simulink model "Pojednostavljeni_model_backstepping"  (R2020b)
settings: Solver=ode4  StartTime=0.0  StopTime=1000  FixedStep=0.01  RelTol=1e-3
model workspace (MAT data in the model file):
  D1 = 0
  D2 = 0
  D3 = 0
  Kd1 = 0
  Kd2 = 0
  Kd3 = 0
  Kp1 = 0
  Kp2 = 0
  Kp3 = 0
undefined symbols (not defined in the file): B, D, E_c, gama_c, gama_vjet, H, Iz, KD1, KD2, KD3, KP1, KP2, KP3, Kurs_poc, L, La1, La2, La3, m, N_c, Nr, Nrdot, Nv, Polozaj_poc_E, Polozaj_poc_N, r_o, ro, ro_vj, Sig, T, V_c, V_vj, Xu, Xudot, Yr, Yrdot, Yv, Yvdot
libraries: simulink_extras x9, simulink x2
settings Model: Creator=Luka  LastModifiedBy=Luka
settings SolverCC: AlgebraicLoopSolver=LineSearch

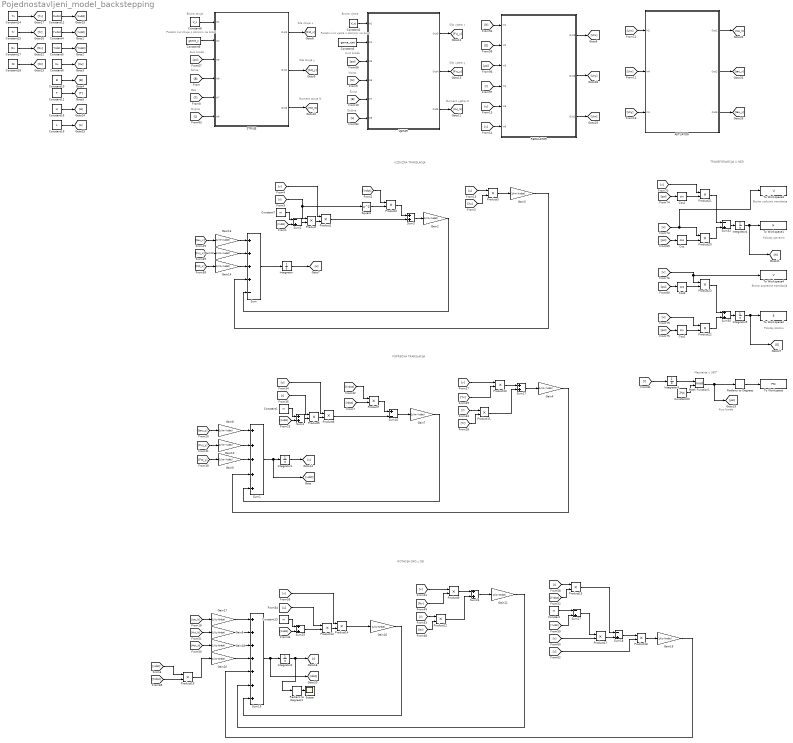
== system Pojednostavljeni_model_backstepping ==
  note: Mapiranje u 360°
  note: Duljina
  note: Visina
  note: Gaz
  note: Širina
  note: Kurs broda
  note: Sila struje x
  note: Kurs broda
  note: Pocetni kut struje s obzirom na brod
  note: Brzina struje
  note: Brzina vjetra
  note: Pocetni kut vjetra s obzirom na brod
  note: Kurs broda
  note: Sila vjetra x
  note: Sila vjetra y
  note: Moment vjetra N
  note: Sila struje y
  note: Moment struje N
  note: UZDUŽNA TRANSLACIJA
  note: POPREČNA TRANSLACIJA
  note: ROTACIJA OKO z OSI
  note: TRANSFORAMCIJA U NED
  note: Položaj istočno
  note: Položaj sjeverno
  note: Brzina uzdužna translacija
  note: Brzina poprečna translacija
  note: Širina
  note: Duljina
  AKTUATOR : Subsystem
  Constant{,1,7,13} (4 alike) : Constant  Value=m
  Constant10 : Constant  Value=B
  Constant11 : Constant  Value=T
  Constant12 : Constant  Value=Xudot
  Constant14 : Constant  Value=Yv
  Constant15 : Constant  Value=Yr
  Constant16 : Constant  Value=H
  Constant17 : Constant  Value=Nv
  Constant18 : Constant  Value=Nr
  Constant19 : Constant  Value=L
  Constant2 : Constant  Value=V_vj
  Constant20 : Constant  Value=2*pi
  Constant3 : Constant  Value=gama_vjet
  Constant4 : Constant  Value=Yvdot
  Constant5 : Constant  Value=Yrdot
  Constant6 : Constant  Value=Xu
  Constant8 : Constant  Value=V_c
  Constant9 : Constant  Value=gama_c
  Cos : Trigonometry  Operator=cos
  Cos1 : Trigonometry
  Cos2 : Trigonometry
  Cos3 : Trigonometry  Operator=cos
  Gain{4,7..10} (5 alike) : Gain  Gain=1/(m-Yvdot)
  Gain{5,11,16..20} (7 alike) : Gain  Gain=1/(Iz-Nrdot)
  Gain{2..3,12..14} (5 alike) : Gain  Gain=1/(m-Xudot)
  Integrator : Integrator
  Integrator1 : Integrator
  Integrator2 : Integrator
  Integrator3 : Integrator  InitialCondition=Kurs_poc
  Integrator4 : Integrator  InitialCondition=Polozaj_poc_N
  Integrator5 : Integrator  InitialCondition=Polozaj_poc_E
  Math Function1 : Math  Operator=mod  SaturateOnIntegerOverflow=on
  Product{,1..3,5..7,9..15,17..23} (21 alike) : Product
  REGULATOR : Subsystem
  Radians to Degrees : simulink_extras/Transformations/Radians to Degrees
  Radians to Degrees1 : simulink_extras/Transformations/Radians to Degrees
  STRUJE : Subsystem
  Scope : Scope
  Square : Math  Operator=square  SaturateOnIntegerOverflow=on
  Sum : Sum  Inputs=++++-
  Sum1 : Sum  Inputs=+++++
  Sum10 : Sum  Inputs=+-
  Sum15 : Sum  Inputs=+++++++
  Sum{3..4,17,24..25,35} (6 alike) : Sum
  Sum{2,18,27,32} (4 alike) : Sum  Inputs=-+
  To Workspace : ToWorkspace  VariableName=PSI  SaveFormat=Timeseries  SampleTime=-1
  To Workspace1 : ToWorkspace  VariableName=N  SaveFormat=Timeseries  SampleTime=-1
  To Workspace2 : ToWorkspace  VariableName=E  SaveFormat=Timeseries  SampleTime=-1
  To Workspace3 : ToWorkspace  VariableName=U  SaveFormat=Timeseries  SampleTime=-1
  To Workspace4 : ToWorkspace  VariableName=V  SaveFormat=Timeseries  SampleTime=-1
  VJETAR : Subsystem
  wires:
  Constant2/1 -> VJETAR/1(In1)
  Constant3/1 -> VJETAR/2(In2)
  [psi] -> VJETAR/3(In5)
  VJETAR/1(Out3) -> [Fvj_x]
  VJETAR/2(Out4) -> [Fvj_y]
  VJETAR/3(Out5) -> [Mvj_N]
  Sum/1 -> Integrator/1
  Constant4/1 -> [Yvdot]
  Constant5/1 -> [Yrdot]
  Constant6/1 -> [Xu]
  Constant7/1 -> Sum2/1
  Sum2/1 -> Product/2
  [r] -> Square/1, Product/1
  [Yvdot] -> Sum2/2
  Constant8/1 -> STRUJE/1(In1)
  [psi] -> STRUJE/3(In5)
  Constant10/1 -> [B]
  Constant11/1 -> [T]
  [B] -> STRUJE/4(In6)
  [T] -> STRUJE/5(In7)
  [H] -> VJETAR/4(In6)
  [B] -> VJETAR/5(In7)
  Product/1 -> Product1/2
  Product1/1 -> Sum3/2
  Square/1 -> Product2/2
  [Yrdot] -> Product2/1
  Product2/1 -> Sum3/1
  Integrator/1 -> [u]
  [v] -> Product1/1
  [u] -> Product3/1
  [Xu] -> Product3/2
  Gain2/1 -> Sum/5
  [Fst_y] -> Gain9/1
  Gain7/1 -> Sum1/5
  Product6/1 -> Sum10/2
  Gain10/1 -> Sum1/2
  Sum10/1 -> Gain7/1
  Product5/1 -> Product6/2
  [r] -> Product5/1
  [Yrdot] -> Product7/1
  [Fvj_y] -> Gain10/1
  [u] -> Product6/1
  Product7/1 -> Sum10/1
  Gain9/1 -> Sum1/3
  Gain8/1 -> Sum1/1
  Integrator1/1 -> [v]
  [Xudot] -> Sum4/2
  Constant1/1 -> Sum4/1
  Sum4/1 -> Product5/2
  Product3/1 -> Gain3/1
  Gain13/1 -> Sum/1
  Gain12/1 -> Sum/2
  Gain14/1 -> Sum/3
  [Fvj_x] -> Gain12/1
  Sum3/1 -> Gain2/1
  Constant12/1 -> [Xudot]
  [rdot] -> Product7/2
  [v] -> Product10/1
  [Yv] -> Product10/2
  Product10/1 -> Sum17/1
  [r] -> Product11/1
  [Yr] -> Product11/2
  Product11/1 -> Sum17/2
  Constant14/1 -> [Yv]
  Constant15/1 -> [Yr]
  Gain4/1 -> Sum1/4
  Gain16/1 -> Sum15/7
  Gain18/1 -> Sum15/3
  [Mvj_N] -> Gain5/1
  Product14/1 -> Gain16/1
  Gain11/1 -> Sum15/6
  Integrator2/1 -> Radians to Degrees1/1, [r]
  Product12/1 -> Sum24/2
  [r] -> Product12/1
  Gain5/1 -> Sum15/2
  [Nr] -> Product12/2
  Sum25/1 -> Product13/2
  [Xudot] -> Sum25/2
  Constant13/1 -> Sum25/1
  Gain17/1 -> Sum15/1
  [v] -> Product9/1
  [Nv] -> Product9/2
  [u] -> Product13/1
  Product9/1 -> Sum24/1
  Sum15/1 -> Integrator2/1, [rdot]
  [Mst_N] -> Gain18/1
  Product13/1 -> Product14/2
  [v] -> Product14/1
  Constant17/1 -> [Nv]
  Constant18/1 -> [Nr]
  [r] -> Product15/1
  [Yrdot] -> Product15/2
  Product15/1 -> Sum18/1
  Constant/1 -> Sum27/1
  [Yvdot] -> Sum27/2
  [v] -> Product17/2
  Sum27/1 -> Product17/1
  Product17/1 -> Sum18/2
  Sum18/1 -> Product18/1
  Product18/1 -> Gain19/1
  Gain19/1 -> Sum15/5
  [Yrdot] -> Product19/2
  [vdot] -> Product19/1
  Product19/1 -> Gain20/1
  Gain20/1 -> Sum15/4
  Product20/1 -> Sum32/2
  [psi] -> Cos/1
  Cos/1 -> Product20/2
  [u] -> To Workspace3/1, Product20/1
  Cos1/1 -> Product21/2
  [psi] -> Cos1/1
  [v] -> Product21/1
  Product21/1 -> Sum32/1
  Sum32/1 -> Integrator4/1
  Integrator4/1 -> [N], To Workspace1/1
  Cos3/1 -> Product23/2
  Product22/1 -> Sum35/2
  Product23/1 -> Sum35/1
  [u] -> Product22/1
  [psi] -> Cos2/1
  Sum35/1 -> Integrator5/1
  Cos2/1 -> Product22/2
  [psi] -> Cos3/1
  [r] -> Integrator3/1
  [v] -> Product23/1, To Workspace4/1
  Constant9/1 -> STRUJE/2(In2)
  Constant16/1 -> [H]
  Constant19/1 -> [L]
  [L] -> VJETAR/6(In8)
  [L] -> STRUJE/6(In8)
  Integrator5/1 -> [E], To Workspace2/1
  Radians to Degrees/1 -> To Workspace/1
  Sum17/1 -> Gain4/1
  Sum1/1 -> [vdot], Integrator1/1
  Sum24/1 -> Gain11/1
  [u] -> Product18/2
  Integrator3/1 -> Math Function1/1
  Constant20/1 -> Math Function1/2
  Math Function1/1 -> [psi], Radians to Degrees/1
  [Fst_x] -> Gain14/1
  STRUJE/1(Out3) -> [Fst_x]
  STRUJE/2(Out4) -> [Fst_y]
  STRUJE/3(Out5) -> [Mst_N]
  [tau_x] -> Gain13/1
  [tau_N] -> Gain17/1
  Gain3/1 -> Sum/4
  [tau_y] -> Gain8/1
  AKTUATOR/3(Out6) -> [tau_y]
  AKTUATOR/1(Out1) -> [tau_N]
  [Urn] -> AKTUATOR/1(In2)
  [Urx] -> AKTUATOR/2(In4)
  [E] -> REGULATOR/2(In2)
  REGULATOR/2(Out5) -> [Ury]
  [psi] -> REGULATOR/3(In3)
  [r] -> REGULATOR/4(In4)
  [N] -> REGULATOR/1(In1)
  REGULATOR/1(Out3) -> [Urx]
  AKTUATOR/2(Out2) -> [tau_x]
  [u] -> REGULATOR/5(In5)
  [v] -> REGULATOR/6(In6)
  REGULATOR/3(Out1) -> [Urn]
  [Ury] -> AKTUATOR/3(In1)
  Radians to Degrees1/1 -> Scope/1

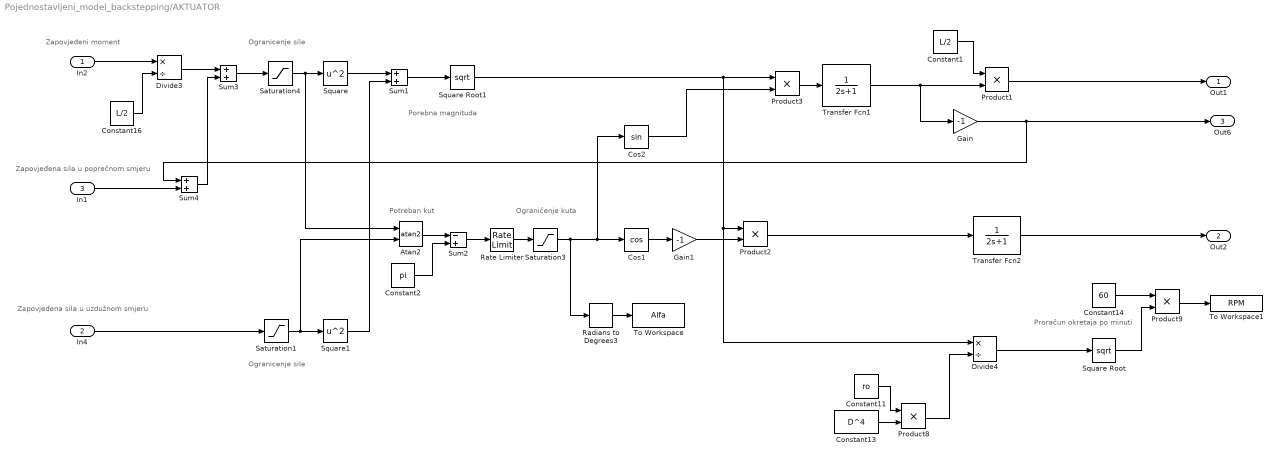
== system Pojednostavljeni_model_backstepping/AKTUATOR ==
  note: Zapovjeđena sila u poprečnom smjeru
  note: Porebna magnituda
  note: Zapovjeđeni moment
  note: Zapovjeđena sila u uzdužnom smjeru
  note: Proračun okretaja po minuti
  note: Ograničenje kuta
  note: Ogranicenje sile
  note: Potreban kut
  note: Ogranicenje sile
  In2 : Inport
  In4 : Inport  Port=2
  In1 : Inport  Port=3
  Atan2 : Trigonometry  Operator=atan2
  Constant1 : Constant  Value=L/2
  Constant11 : Constant  Value=ro
  Constant13 : Constant  Value=D^4
  Constant14 : Constant  Value=60
  Constant16 : Constant  Value=L/2
  Constant2 : Constant  Value=pi
  Cos1 : Trigonometry  Operator=cos
  Cos2 : Trigonometry
  Divide3 : Product  Inputs=*/
  Divide4 : Product  Inputs=*/
  Gain : Gain  Gain=-1
  Gain1 : Gain  Gain=-1
  Product{1..3,8..9} (5 alike) : Product
  Radians to Degrees3 : simulink_extras/Transformations/Radians to Degrees
  Rate Limiter : RateLimiter  RisingSlewLimit=40*pi/180  FallingSlewLimit=-40*pi/180  SampleTimeMode=inherited
  Saturation1 : Saturate  UpperLimit=300  LowerLimit=0
  Saturation3 : Saturate  UpperLimit=250*pi/180  LowerLimit=110*pi/180
  Saturation4 : Saturate  UpperLimit=280  LowerLimit=-280
  Square : Math  Operator=square  SaturateOnIntegerOverflow=on
  Square Root : Sqrt  SaturateOnIntegerOverflow=on
  Square Root1 : Sqrt  SaturateOnIntegerOverflow=on
  Square1 : Math  Operator=square  SaturateOnIntegerOverflow=on
  Sum1 : Sum
  Sum2 : Sum  Inputs=-+
  Sum3 : Sum
  Sum4 : Sum
  To Workspace : ToWorkspace  VariableName=Alfa  SaveFormat=Timeseries  SampleTime=-1
  To Workspace1 : ToWorkspace  VariableName=RPM  SaveFormat=Timeseries  SampleTime=-1
  Transfer Fcn1 : TransferFcn  Denominator=[2 1]
  Transfer Fcn2 : TransferFcn  Denominator=[2 1]
  Out1 : Outport
  Out2 : Outport  Port=2
  Out6 : Outport  Port=3
  wires:
  Sum2/1 -> Rate Limiter/1
  Product8/1 -> Divide4/2
  Gain/1 -> Sum4/1, Out6/1
  Sum1/1 -> Square Root1/1
  Constant16/1 -> Divide3/2
  Saturation3/1 -> Cos2/1, Cos1/1, Radians to Degrees3/1
  Saturation4/1 -> Atan2/1, Square/1
  Divide3/1 -> Sum3/1
  Cos1/1 -> Gain1/1
  Gain1/1 -> Product2/2
  In4/1 -> Saturation1/1
  Constant11/1 -> Product8/1
  Rate Limiter/1 -> Saturation3/1
  Transfer Fcn1/1 -> Gain/1, Product1/2
  Square1/1 -> Sum1/2
  Square/1 -> Sum1/1
  Product3/1 -> Transfer Fcn1/1
  Cos2/1 -> Product3/2
  Atan2/1 -> Sum2/1
  In2/1 -> Divide3/1
  Product2/1 -> Transfer Fcn2/1
  Product9/1 -> To Workspace1/1
  Product1/1 -> Out1/1
  Square Root/1 -> Product9/2
  Transfer Fcn2/1 -> Out2/1
  Constant13/1 -> Product8/2
  Divide4/1 -> Square Root/1
  Square Root1/1 -> Divide4/1, Product2/1, Product3/1
  Saturation1/1 -> Atan2/2, Square1/1
  Radians to Degrees3/1 -> To Workspace/1
  Constant2/1 -> Sum2/2
  Constant1/1 -> Product1/1
  Constant14/1 -> Product9/1
  Sum3/1 -> Saturation4/1
  In1/1 -> Sum4/2
  Sum4/1 -> Sum3/2

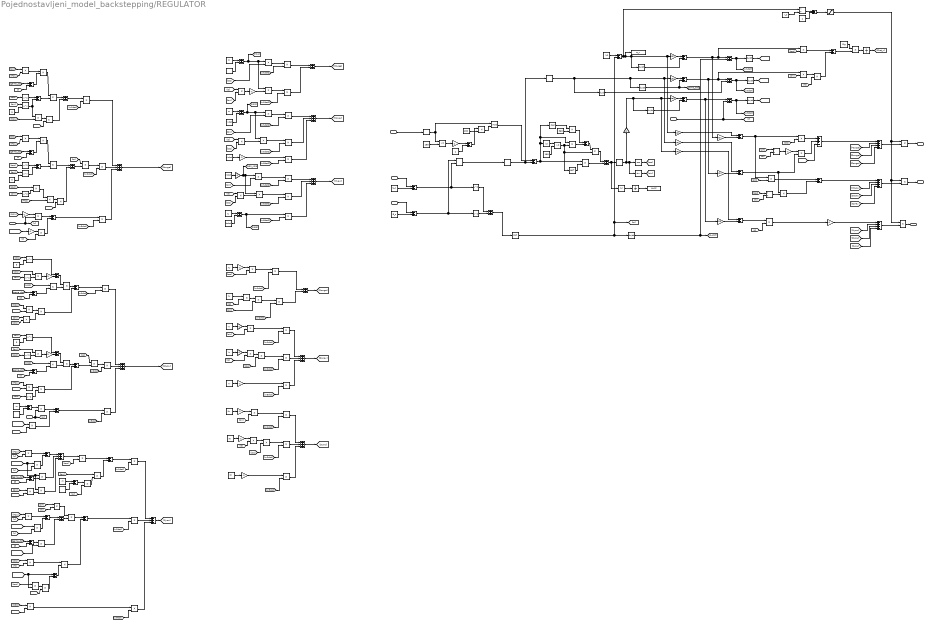
== system Pojednostavljeni_model_backstepping/REGULATOR ==
  note: Integralno djelovanje u napredovanju
  note: Zapovjeđeni moment
  note: Dx33
  note: Dx32
  note: Dx31
  note: Dx12
  note: Dx11
  note: Cx32
  note: Cx31
  note: Cx13
  note: Cx21
  note: v
  note: u
  note: Cx11
  note: Mx11
  note: xr1dot
  note: r
  note: z13dot
  note: z12dot
  note: z11dot
  note: x1dot
  note: z13
  note: z11
  note: x1d
  note: Kurs u +/- 180°(x3)
  note: Udaljenost od centra kruznice (x1)
  note: Pogreška kuta -/+ 180
  note: Zapovjeđena sila u uzdužnom smjeru
  note: Zapovjeđena sila u poprečnom smjeru
  note: Kurs broda
  note: Potreban kurs broda +/- 180
  note: Polozaj N
  note: Polozaj E
  note: Polozaj kruznice N
  note: Polozaj kruznice E
  note: z12
  note: x3dot
  note: x2dot
  note: z21
  note: z22
  note: z23
  note: xr2dot
  note: xr3dot
  note: xr1dot2
  note: xr2dot2
  note: xr3dot2
  note: Mx12
  note: Mx21
  note: Mx22
  note: Mx23
  note: Mx31
  note: Mx32
  note: Mx33
  note: Cx12
  note: Cx22
  note: Cx23
  note: Cx33
  note: Dx21
  note: Dx22
  note: Dx23
  note: Ublažavanje regulacije u slučaju da je brod unutar kružnice
  In1 : Inport
  In2 : Inport  Port=2
  In3 : Inport  Port=3
  In4 : Inport  Port=4
  In5 : Inport  Port=5
  In6 : Inport  Port=6
  Abs : Abs
  Abs3 : Abs
  Atan2 : Trigonometry  Operator=atan2
  Constant : Constant  Value=r_o
  Constant1 : Constant  Value=N_c
  Constant10 : Constant  Value=Yrdot
  Constant12 : Constant  Value=Iz
  Constant13 : Constant  Value=Nrdot
  Constant14 : Constant  Value=180
  Constant{15..16,19..20} (4 alike) : Constant  Value=3
  Constant17 : Constant  Value=180
  Constant18 : Constant
  Constant2 : Constant  Value=E_c
  Constant{3,6,21,23} (4 alike) : Constant  Value=m
  Constant22 : Constant  Value=Xudot
  Constant24 : Constant  Value=Xudot
  Constant25 : Constant  Value=180
  Constant26 : Constant  Value=Xu
  Constant27 : Constant  Value=360
  Constant28 : Constant  Value=Xu
  Constant29 : Constant  Value=Yv
  Constant30 : Constant  Value=Yv
  Constant31 : Constant  Value=Yr
  Constant32 : Constant  Value=Nv
  Constant33 : Constant  Value=Nv
  Constant34 : Constant  Value=Nr
  Constant39 : Constant  Value=r_o
  Constant4 : Constant  Value=Xudot
  Constant40 : Constant
  Constant5 : Constant  Value=Sig
  Constant7 : Constant  Value=Yvdot
  Constant9 : Constant  Value=Yrdot
  Cos : Trigonometry  Operator=cos
  Degrees to Radians : simulink_extras/Transformations/Degrees to Radians
  Degrees to Radians1 : simulink_extras/Transformations/Degrees to Radians
  Derivative{,1..7} (8 alike) : Derivative
  Divide : Product  Inputs=*/
  Divide1 : Product  Inputs=*/
  Divide2 : Product  Inputs=*/
  Gain : Gain  Gain=La1
  Gain1 : Gain  Gain=La3
  Gain{7..11,14..20,24,27..28} (15 alike) : Gain  Gain=-1
  Gain12 : Gain  Gain=3
  Gain13 : Gain  Gain=3
  Gain2 : Gain  Gain=La2
  Gain21 : Gain  Gain=KD1
  Gain22 : Gain  Gain=KD3
  Gain23 : Gain  Gain=KD2
  Gain3 : Gain  Gain=KP1
  Gain4 : Gain  Gain=KP3
  Gain5 : Gain  Gain=2
  Gain6 : Gain  Gain=KP2
  GreaterThan : RelationalOperator  OutDataTypeStr=boolean  RndMeth=Simplest
  GreaterThan1 : RelationalOperator  OutDataTypeStr=boolean  RndMeth=Simplest
  Integrator : Integrator
  Integrator1 : Integrator
  Mod2 : Math  Operator=mod  SaturateOnIntegerOverflow=on
  NOT : Logic  Operator=NOT  IconShape=distinctive  AllPortsSameDT=off  OutDataTypeStr=boolean
  Power{,1..3} (4 alike) : Math  Operator=pow  SaturateOnIntegerOverflow=on
  Product{,1..102,104..106} (106 alike) : Product
  Radians to Degrees : simulink_extras/Transformations/Radians to Degrees
  Radians to Degrees2 : simulink_extras/Transformations/Radians to Degrees
  Saturation : Saturate  UpperLimit=1  LowerLimit=0
  Sign : Signum
  Sin : Trigonometry
  Sqrt : Sqrt  SaturateOnIntegerOverflow=on
  Square{,1..7} (8 alike) : Math  Operator=square  SaturateOnIntegerOverflow=on
  Sum{,1,5,7..10,14,17,29,32,43,59} (13 alike) : Sum  Inputs=-+
  Sum{11..13,20..22,24..26,28,31,36..37,39,41..42,44} (17 alike) : Sum  Inputs=+-
  Sum{2..4,6,15,18,23,30,33,35,40,45..46,48,51..53,55,64} (19 alike) : Sum
  Sum{16,19,27,34,47,49..50} (7 alike) : Sum  Inputs=+++
  Sum38 : Sum  Inputs=+-+
  Sum54 : Sum  Inputs=++-
  Sum56 : Sum  Inputs=++++
  Sum57 : Sum  Inputs=++++
  Sum58 : Sum  Inputs=++++
  To Workspace : ToWorkspace  VariableName=e_psi  SaveFormat=Timeseries  SampleTime=-1
  To Workspace1 : ToWorkspace  VariableName=e_x  SaveFormat=Timeseries  SampleTime=-1
  Out3 : Outport
  Out5 : Outport  Port=2
  Out1 : Outport  Port=3
  wires:
  Constant1/1 -> Sum/2
  In1/1 -> Sum/1
  Constant2/1 -> Sum1/2
  In2/1 -> Sum1/1
  Sum1/1 -> Square/1, Atan2/1
  Sum/1 -> Square1/1, Atan2/2
  Square1/1 -> Sum2/1
  Square/1 -> Sum2/2
  Sum2/1 -> Sqrt/1
  Atan2/1 -> Radians to Degrees2/1
  Radians to Degrees2/1 -> Degrees to Radians1/1, Sum8/2
  Constant18/1 -> Sum14/2
  Gain5/1 -> Sum14/1
  Radians to Degrees/1 -> GreaterThan/1, Mod2/1
  Constant17/1 -> GreaterThan/2
  GreaterThan/1 -> Gain5/1
  Sum14/1 -> Product10/1
  Mod2/1 -> Sum8/1
  Constant14/1 -> Product10/2
  Product10/1 -> Mod2/2
  Abs3/1 -> GreaterThan1/1
  Constant25/1 -> GreaterThan1/2
  GreaterThan1/1 -> Product16/2, NOT/1, Product15/2
  Sum8/1 -> Product15/1, Sign/1, Abs3/1, Product18/1
  Product15/1 -> Sum17/2
  Sum17/1 -> Product16/1
  Product16/1 -> Sum18/1
  Constant27/1 -> Product17/2
  Product17/1 -> Sum17/1
  NOT/1 -> Product18/2
  Product18/1 -> Sum18/2
  Sign/1 -> Product17/1
  Constant/1 -> Sum5/1
  Derivative1/1 -> Sum3/2
  Derivative2/1 -> Sum4/2, [gama_dot]
  Derivative/1 -> [ro_dot], Sum7/2
  Gain/1 -> Sum3/1
  Gain2/1 -> Sum4/1
  Gain1/1 -> Sum6/1
  Sum4/1 -> Gain23/1, Product100/1, Sum9/1
  Sum7/1 -> [xr1dot], Derivative4/1
  Sum9/1 -> [xr2dot], Derivative5/1
  Sum10/1 -> [xr3dot], Derivative6/1
  Constant3/1 -> Sum11/1
  Constant4/1 -> Sum11/2
  Sum11/1 -> [M11], Product1/1, Product3/1
  Cos/1 -> [cos]
  Sin/1 -> [sin]
  [cos] -> Product1/2
  [ro] -> Product2/1
  [sin] -> Product2/2
  Product2/1 -> Gain7/1
  Gain7/1 -> Product3/2
  Constant7/1 -> Sum12/2
  Constant6/1 -> Sum12/1
  Sum12/1 -> [M22], Product6/1, Product4/1
  [sin] -> Product4/2
  [ro] -> Product5/1
  [cos] -> Product5/2
  Product5/1 -> Product6/2
  Constant9/1 -> Gain8/1
  [sin] -> Product7/2
  Constant10/1 -> Gain9/1
  Gain9/1 -> [M32_M23], Product9/1, Product7/1
  [ro] -> Product8/1
  Product8/1 -> Product9/2
  [cos] -> Product8/2
  Constant12/1 -> Sum13/1
  Constant13/1 -> Sum13/2
  Derivative4/1 -> [xr1dot2]
  Derivative5/1 -> [xr2dot2]
  Derivative6/1 -> [xr3dot2]
  Product1/1 -> Product/1
  [xr1dot2] -> Product/2
  Product3/1 -> Product11/1
  [xr2dot2] -> Product11/2
  Product11/1 -> Sum15/2
  Product/1 -> Sum15/1
  Product4/1 -> Product12/1
  [xr1dot2] -> Product12/2
  [xr2dot2] -> Product13/2
  Product6/1 -> Product13/1
  Gain8/1 -> Product14/1
  Product12/1 -> Sum16/1
  Product13/1 -> Sum16/2
  [xr3dot2] -> Product14/2
  Product14/1 -> Sum16/3
  Product7/1 -> Product19/1
  [xr1dot2] -> Product19/2
  Product9/1 -> Product20/1
  [xr2dot2] -> Product20/2
  Sum13/1 -> [M33], Product21/1
  [xr3dot2] -> Product21/2
  Product20/1 -> Sum19/2
  Product21/1 -> Sum19/3
  [sin] -> Product22/1
  [M11] -> Product22/2
  [gama_dot] -> Sum20/1
  In4/1 -> Sum10/2, [r]
  [r] -> Sum20/2
  Product22/1 -> Product23/1
  Sum20/1 -> Product23/2
  [cos] -> Square2/1
  Square2/1 -> Sum21/1
  [sin] -> Power/1
  Constant15/1 -> Power/2
  Power/1 -> Product25/1, Sum21/2
  Sum21/1 -> Product24/2
  Product23/1 -> Product24/1
  Product24/1 -> Sum22/1
  [M11] -> Product25/2
  Product25/1 -> Product26/1
  [ro_dot] -> Product26/2
  Product26/1 -> Sum22/2
  Sum22/1 -> Product27/1
  [xr1dot] -> Product27/2
  Product27/1 -> Sum27/1
  [M11] -> Product31/2
  Product29/1 -> Product30/1
  Product31/1 -> Product32/1
  [sin] -> Power1/1
  [cos] -> Product28/1
  Product28/1 -> Product29/1
  Constant16/1 -> Power1/2
  [r] -> Sum24/2
  Sum25/1 -> Product30/2
  [ro_dot] -> Product32/2
  Sum24/1 -> Product29/2
  [M11] -> Product28/2
  Square3/1 -> Sum25/1
  Product32/1 -> Sum26/2
  [cos] -> Square3/1
  Sum26/1 -> Product34/2
  Power1/1 -> Sum25/2
  Product30/1 -> Sum26/1
  [xr2dot] -> Product33/2
  [gama_dot] -> Sum24/1
  Product33/1 -> Sum27/2
  [ro] -> Product34/1
  Product34/1 -> Product33/1
  [sin] -> Square4/1
  [cos] -> Product35/1
  Square4/1 -> Product35/2
  Product35/1 -> Product31/1
  [M11] -> Gain10/1
  In6/1 -> [v], Product36/2
  Gain10/1 -> Product36/1
  Product36/1 -> Sum23/1
  [M32_M23] -> Gain11/1
  Gain11/1 -> Product37/1
  [r] -> Product37/2
  Product37/1 -> Sum23/2
  [r] -> Sum28/2
  Sum28/1 -> Product38/2
  [gama_dot] -> Sum28/1
  [M22] -> Product38/1
  Product38/1 -> Product39/2
  [cos] -> Product43/1
  Product39/1 -> Sum30/1
  [M22] -> Product40/1
  [ro_dot] -> Product40/2
  Product40/1 -> Product41/1
  Product41/1 -> Sum30/2
  [sin] -> Product42/1
  [cos] -> Product42/2
  Product42/1 -> Product41/2
  [sin] -> Square5/1
  Square5/1 -> Product43/2
  Product43/1 -> Gain12/1
  Gain12/1 -> Sum29/2
  [cos] -> Power2/1
  Constant19/1 -> Power2/2
  Power2/1 -> Sum29/1
  Sum29/1 -> Product39/1
  Sum30/1 -> Product44/1
  [xr1dot] -> Product44/2
  Gain13/1 -> Sum32/2
  Square7/1 -> Product48/2
  [M22] -> Product47/1
  [M22] -> Product45/1
  Power3/1 -> Sum32/1
  Constant20/1 -> Power3/2
  [gama_dot] -> Sum31/1
  Product46/1 -> Sum33/1
  [r] -> Sum31/2
  [xr2dot] -> Product51/2
  [sin] -> Product50/1
  Sum31/1 -> Product45/2
  [ro_dot] -> Product47/2
  Product47/1 -> Product48/1
  Product48/1 -> Sum33/2
  Sum32/1 -> Product46/1
  Product45/1 -> Product46/2
  [sin] -> Power3/1
  Square6/1 -> Product50/2
  Product50/1 -> Gain13/1
  [cos] -> Square7/1
  [cos] -> Square6/1
  Sum33/1 -> Product52/2
  Product52/1 -> Product51/1
  [ro] -> Product52/1
  Product44/1 -> Sum34/1
  Product51/1 -> Sum34/2
  Product49/1 -> Sum27/3
  [xr3dot] -> Product49/2
  Sum23/1 -> Product49/1
  Constant21/1 -> Sum35/1
  Constant22/1 -> Sum35/2
  Sum35/1 -> Product53/1
  In5/1 -> [u], Product53/2
  Product53/1 -> Sum36/1
  [M32_M23] -> Product54/1
  [ro_dot] -> Product54/2
  Product54/1 -> Sum36/2
  Sum36/1 -> Product55/1
  [xr3dot] -> Product55/2
  Product55/1 -> Sum34/3
  [v] -> Product56/2
  [M22] -> Product56/1
  Product56/1 -> Sum37/1
  [r] -> Product57/2
  Product57/1 -> Sum37/2
  Sum37/1 -> Sum38/1
  [cos] -> Product58/2
  [r] -> Sum39/2
  Sum39/1 -> Product59/2
  [gama_dot] -> Sum39/1
  Product59/1 -> Sum38/2
  Sum38/1 -> Product58/1
  [M32_M23] -> Product57/1, Product61/1, Product59/1
  [ro_dot] -> Product60/2
  [sin] -> Product60/1
  Product60/1 -> Product61/2
  Product61/1 -> Sum38/3
  Product58/1 -> Sum40/1
  Product62/1 -> Product63/2
  Constant23/1 -> Sum41/1
  Sum41/1 -> Product62/1
  Constant24/1 -> Sum41/2
  [u] -> Product62/2
  [sin] -> Product63/1
  Product63/1 -> Sum40/2
  Sum40/1 -> Product64/1
  [xr1dot] -> Product64/2
  [sin] -> Product65/1
  Product65/1 -> Product69/1
  [ro] -> Product65/2
  Product66/1 -> Sum42/1
  [v] -> Product66/2
  Product67/1 -> Sum42/2
  Sum42/1 -> Sum43/1
  [M22] -> Product66/1
  [r] -> Product67/2
  [M32_M23] -> Product67/1
  [gama_dot] -> Sum44/1
  [r] -> Sum44/2
  Sum44/1 -> Product68/1
  [M32_M23] -> Product68/2
  Product68/1 -> Sum43/2
  Sum43/1 -> Product69/2
  [ro] -> Product70/2
  [cos] -> Product70/1
  Product69/1 -> Sum45/1
  Product70/1 -> Product71/1
  Product71/1 -> Sum45/2
  [M32_M23] -> Sum46/1, Product72/2
  [cos] -> Product72/1
  [ro_dot] -> Product73/2
  Product72/1 -> Product73/1
  Product73/1 -> Sum46/2
  Sum46/1 -> Product71/2
  Sum45/1 -> Product74/1
  [xr2dot] -> Product74/2
  Product64/1 -> Sum47/1
  Product74/1 -> Sum47/2
  [M33] -> Product75/1
  [ro_dot] -> Product75/2
  [xr3dot] -> Product76/2
  Product75/1 -> Product76/1
  Product76/1 -> Sum47/3
  Constant26/1 -> Gain14/1
  [cos] -> Product77/2
  Gain14/1 -> Product77/1
  Product77/1 -> Product78/1
  [xr1dot] -> Product78/2
  Product78/1 -> Sum48/1
  Constant28/1 -> Product79/1
  [ro] -> Product79/2
  Product79/1 -> Product80/1
  [sin] -> Product80/2
  [xr2dot] -> Product81/2
  Product80/1 -> Product81/1
  Product81/1 -> Sum48/2
  Constant29/1 -> Gain15/1
  Gain15/1 -> Product82/1
  [sin] -> Product82/2
  Product82/1 -> Product83/1
  [xr1dot] -> Product83/2
  Constant30/1 -> Gain16/1
  Gain16/1 -> Product84/1
  [ro] -> Product84/2
  Product84/1 -> Product85/1
  [cos] -> Product85/2
  Product85/1 -> Product86/1
  [xr2dot] -> Product86/2
  Constant31/1 -> Gain17/1
  Gain17/1 -> Product87/1
  [xr3dot] -> Product87/2
  Product83/1 -> Sum49/1
  Product86/1 -> Sum49/2
  Product87/1 -> Sum49/3
  Constant32/1 -> Gain18/1
  [sin] -> Product88/2
  Gain18/1 -> Product88/1
  Product88/1 -> Product89/1
  [xr1dot] -> Product89/2
  Constant33/1 -> Gain19/1
  Gain19/1 -> Product90/1
  [ro] -> Product90/2
  Product90/1 -> Product91/1
  [cos] -> Product91/2
  [xr2dot] -> Product92/2
  Product91/1 -> Product92/1
  Product89/1 -> Sum50/1
  Product92/1 -> Sum50/2
  Constant34/1 -> Gain20/1
  Gain20/1 -> Product93/1
  [xr3dot] -> Product93/2
  Product93/1 -> Sum50/3
  Gain3/1 -> Sum51/1
  Gain21/1 -> Sum51/2
  Gain23/1 -> Sum52/2
  Gain6/1 -> Sum52/1
  Gain22/1 -> Sum53/2
  Gain4/1 -> Sum53/1
  [cos] -> Product94/2
  Sum51/1 -> Product96/1, Product94/1
  Product94/1 -> Sum54/1
  [sin] -> Divide/1
  [ro] -> Divide/2
  Divide/1 -> Gain24/1
  Gain24/1 -> Product95/1
  Sum52/1 -> Product97/1, Product95/2
  Product95/1 -> Sum54/2
  [sin] -> Product96/2
  Product96/1 -> Sum55/1
  [cos] -> Divide1/1
  [ro] -> Divide1/2
  Divide1/1 -> Product97/2
  Product97/1 -> Sum55/2
  Sum53/1 -> Product98/1
  [r] -> Product98/2
  Sum15/1 -> [Msurge]
  Sum16/1 -> [Msway]
  Sum19/1 -> [Myaw]
  Sum48/1 -> [Dsurge]
  Sum49/1 -> [Dsway]
  Sum50/1 -> [Dyaw]
  Sum27/1 -> [Csurge]
  Sum34/1 -> [Csway]
  Sum47/1 -> [Cyaw]
  Sum54/1 -> Sum56/1
  [Msurge] -> Sum56/2
  [Dsurge] -> Sum56/3
  [Csurge] -> Sum56/4
  Sum56/1 -> Product104/2
  Sum55/1 -> Sum57/1
  [Msway] -> Sum57/2
  [Dsway] -> Sum57/3
  [Csway] -> Sum57/4
  Gain27/1 -> Sum58/1
  [Myaw] -> Sum58/2
  [Dyaw] -> Sum58/3
  [Cyaw] -> Sum58/4
  Sum58/1 -> Product106/2
  Derivative7/1 -> Sum9/2
  Derivative3/1 -> Sum6/2
  In3/1 -> Radians to Degrees/1
  Product19/1 -> Sum19/1
  Sum18/1 -> Abs/1, Degrees to Radians/1
  Degrees to Radians1/1 -> Derivative2/1, Gain6/1, Gain2/1, Derivative7/1
  Degrees to Radians/1 -> Cos/1, Sin/1, Gain28/1
  Gain28/1 -> Derivative3/1, Gain1/1, Gain4/1
  Abs/1 -> Integrator/1
  Integrator/1 -> To Workspace/1
  Constant5/1 -> Product99/1
  [sin] -> Product100/2
  [cos] -> Product101/2
  Product100/1 -> Product102/1
  [ro] -> Product102/2
  Product101/1 -> Sum59/1
  Product102/1 -> Sum59/2
  Sum59/1 -> Product99/2
  Product99/1 -> Integrator1/1
  Integrator1/1 -> [Fhat_x]
  [Fhat_x] -> Sum54/3
  Sqrt/1 -> [ro], Sum5/2, Derivative/1
  Sum3/1 -> Sum7/1, Product101/1, Gain21/1
  Sum6/1 -> Sum10/1, Gain22/1
  Product106/1 -> Out1/1
  Product104/1 -> Out3/1
  Sum57/1 -> Product105/2
  Product105/1 -> Out5/1
  Product98/1 -> Gain27/1
  Constant40/1 -> Sum64/2
  Sum64/1 -> Saturation/1
  Divide2/1 -> Sum64/1
  Saturation/1 -> Product104/1, Product106/1, Product105/1
  Sum5/1 -> Divide2/1, Gain/1, Gain3/1, Derivative1/1, To Workspace1/1
  Constant39/1 -> Divide2/2

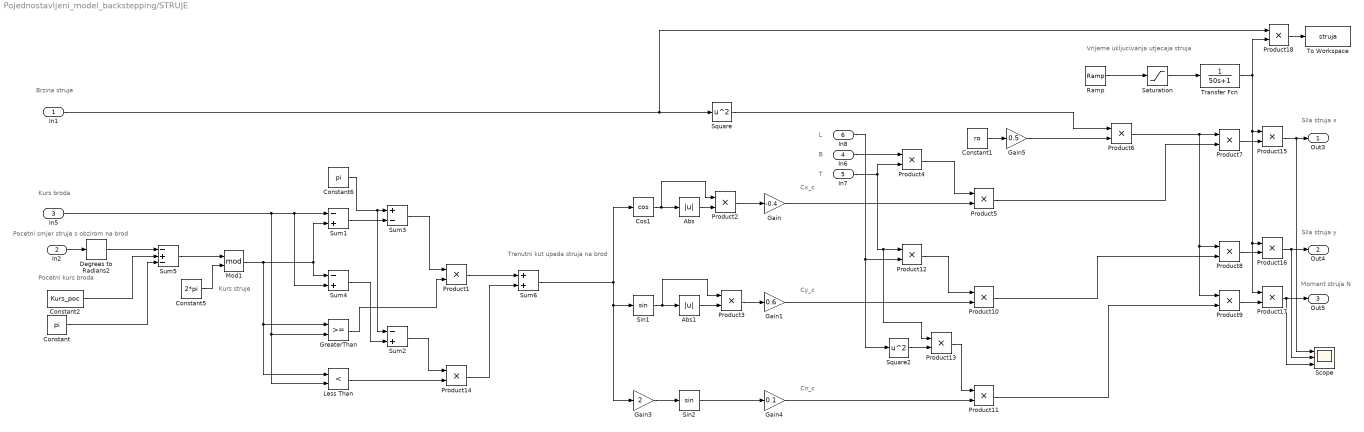
== system Pojednostavljeni_model_backstepping/STRUJE ==
  note: Trenutni kut upada struja na brod
  note: Vrijeme ukljucivanja utjecaja struja
  note: Sila struja x
  note: B
  note: Cx_c
  note: Kurs broda
  note: Pocetni smjer struje s obzirom na brod
  note: Brzina struje
  note: Kurs struje
  note: Cy_c
  note: Cn_c
  note: T
  note: Sila struja y
  note: Moment struja N
  note: L
  note: Pocetni kurs broda
  In1 : Inport
  In2 : Inport  Port=2
  In5 : Inport  Port=3
  In6 : Inport  Port=4
  In7 : Inport  Port=5
  In8 : Inport  Port=6
  Abs : Abs
  Abs1 : Abs
  Constant : Constant  Value=pi
  Constant1 : Constant  Value=ro
  Constant2 : Constant  Value=Kurs_poc
  Constant5 : Constant  Value=2*pi
  Constant6 : Constant  Value=pi
  Cos1 : Trigonometry  Operator=cos
  Degrees to Radians2 : simulink_extras/Transformations/Degrees to Radians
  Gain : Gain  Gain=-0.4
  Gain1 : Gain  Gain=0.6
  Gain3 : Gain  Gain=2
  Gain4 : Gain  Gain=0.1
  Gain5 : Gain  Gain=0.5
  GreaterThan : RelationalOperator  OutDataTypeStr=boolean  RndMeth=Simplest
  Less Than : RelationalOperator  Operator=<  OutDataTypeStr=boolean  RndMeth=Simplest
  Mod1 : Math  Operator=mod  SaturateOnIntegerOverflow=on
  Product{1..18} (18 alike) : Product
  Ramp : simulink/Sources/Ramp  slope=0.002  start=0  InitialOutput=0
  Saturation : Saturate  UpperLimit=1  LowerLimit=-1
  Scope : Scope  NumInputPorts=3
  Sin1 : Trigonometry
  Sin2 : Trigonometry
  Square : Math  Operator=square  SaturateOnIntegerOverflow=on
  Square2 : Math  Operator=square  SaturateOnIntegerOverflow=on
  Sum1 : Sum  Inputs=-+
  Sum2 : Sum  Inputs=-+
  Sum3 : Sum  Inputs=+-
  Sum4 : Sum  Inputs=-+
  Sum5 : Sum  Inputs=-+-
  Sum6 : Sum
  To Workspace : ToWorkspace  VariableName=struja  SaveFormat=Timeseries  SampleTime=-1
  Transfer Fcn : TransferFcn  Denominator=[50 1]
  Out3 : Outport
  Out4 : Outport  Port=2
  Out5 : Outport  Port=3
  wires:
  In1/1 -> Product18/1, Square/1
  Cos1/1 -> Product2/1, Abs/1
  Abs/1 -> Product2/2
  Product2/1 -> Gain/1
  Sin1/1 -> Product3/1, Abs1/1
  Abs1/1 -> Product3/2
  Product3/1 -> Gain1/1
  Gain3/1 -> Sin2/1
  Sin2/1 -> Gain4/1
  Constant1/1 -> Gain5/1
  In6/1 -> Product4/1
  In7/1 -> Product13/1, Product12/1, Product4/2
  Product4/1 -> Product5/1
  Gain5/1 -> Product6/2
  Product6/1 -> Product8/1, Product9/1, Product7/1
  Product7/1 -> Product15/2
  Gain/1 -> Product5/2
  Product5/1 -> Product7/2
  In8/1 -> Product12/2, Square2/1
  Gain1/1 -> Product10/2
  Gain4/1 -> Product11/2
  Product11/1 -> Product9/2
  Product10/1 -> Product8/2
  Product12/1 -> Product10/1
  Square2/1 -> Product13/2
  Product13/1 -> Product11/1
  Constant2/1 -> Sum5/2
  Sum5/1 -> Mod1/1
  In2/1 -> Degrees to Radians2/1
  Degrees to Radians2/1 -> Sum5/1
  Square/1 -> Product6/1
  Constant/1 -> Sum5/3
  Constant5/1 -> Mod1/2
  Mod1/1 -> Sum4/1, Sum1/2, Less Than/1, GreaterThan/1
  In5/1 -> Less Than/2, GreaterThan/2, Sum4/2, Sum1/1
  Constant6/1 -> Sum2/1, Sum3/1
  Sum1/1 -> Sum3/2
  GreaterThan/1 -> Product1/2
  Sum3/1 -> Product1/1
  Less Than/1 -> Product14/2
  Sum4/1 -> Sum2/2
  Sum2/1 -> Product14/1
  Product1/1 -> Sum6/1
  Sum6/1 -> Cos1/1, Gain3/1, Sin1/1
  Product14/1 -> Sum6/2
  Product15/1 -> Scope/1, Out3/1
  Ramp/1 -> Saturation/1
  Product8/1 -> Product16/2
  Product9/1 -> Product17/2
  Product16/1 -> Scope/2, Out4/1
  Product17/1 -> Scope/3, Out5/1
  Saturation/1 -> Transfer Fcn/1
  Transfer Fcn/1 -> Product18/2, Product17/1, Product16/1, Product15/1
  Product18/1 -> To Workspace/1

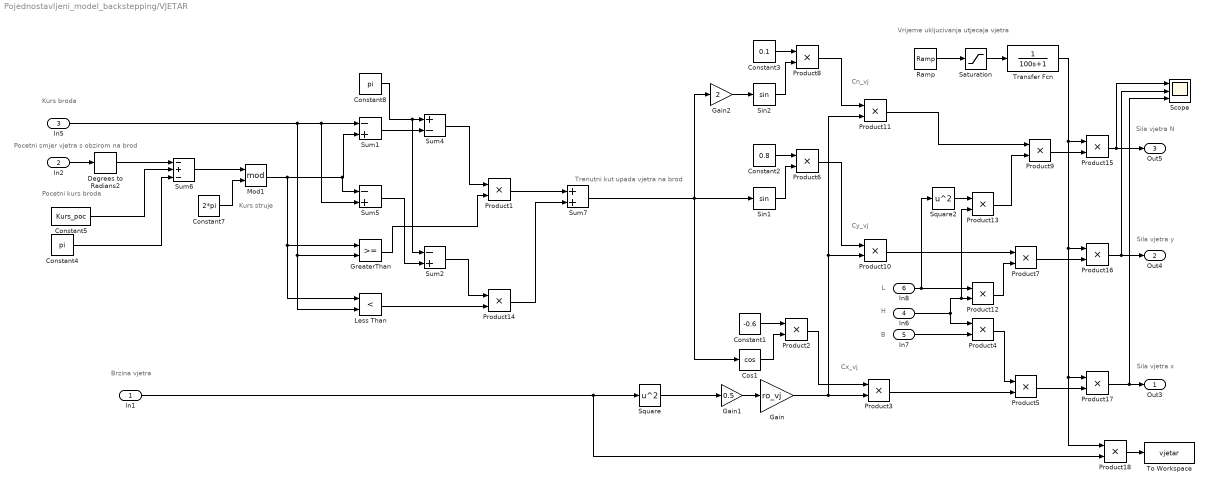
== system Pojednostavljeni_model_backstepping/VJETAR ==
  note: Trenutni kut upada vjetra na brod
  note: Sila vjetra x
  note: H
  note: B
  note: Cx_vj
  note: Brzina vjetra
  note: Cy_vj
  note: Cn_vj
  note: Sila vjetra y
  note: Sila vjetra N
  note: L
  note: Pocetni kurs broda
  note: Kurs broda
  note: Pocetni smjer vjetra s obzirom na brod
  note: Kurs struje
  note: Vrijeme ukljucivanja utjecaja vjetra
  In1 : Inport
  In2 : Inport  Port=2
  In5 : Inport  Port=3
  In6 : Inport  Port=4
  In7 : Inport  Port=5
  In8 : Inport  Port=6
  Constant1 : Constant  Value=-0.6
  Constant2 : Constant  Value=0.8
  Constant3 : Constant  Value=0.1
  Constant4 : Constant  Value=pi
  Constant5 : Constant  Value=Kurs_poc
  Constant7 : Constant  Value=2*pi
  Constant8 : Constant  Value=pi
  Cos1 : Trigonometry  Operator=cos
  Degrees to Radians2 : simulink_extras/Transformations/Degrees to Radians
  Gain : Gain  Gain=ro_vj
  Gain1 : Gain  Gain=0.5
  Gain2 : Gain  Gain=2
  GreaterThan : RelationalOperator  OutDataTypeStr=boolean  RndMeth=Simplest
  Less Than : RelationalOperator  Operator=<  OutDataTypeStr=boolean  RndMeth=Simplest
  Mod1 : Math  Operator=mod  SaturateOnIntegerOverflow=on
  Product{1..18} (18 alike) : Product
  Ramp : simulink/Sources/Ramp  slope=0.002  start=100  InitialOutput=0
  Saturation : Saturate  UpperLimit=1  LowerLimit=0
  Scope : Scope  NumInputPorts=3
  Sin1 : Trigonometry
  Sin2 : Trigonometry
  Square : Math  Operator=square  SaturateOnIntegerOverflow=on
  Square2 : Math  Operator=square  SaturateOnIntegerOverflow=on
  Sum1 : Sum  Inputs=-+
  Sum2 : Sum  Inputs=-+
  Sum4 : Sum  Inputs=+-
  Sum5 : Sum  Inputs=-+
  Sum6 : Sum  Inputs=-+-
  Sum7 : Sum
  To Workspace : ToWorkspace  VariableName=vjetar  SaveFormat=Timeseries  SampleTime=-1
  Transfer Fcn : TransferFcn  Denominator=[100 1]
  Out3 : Outport
  Out4 : Outport  Port=2
  Out5 : Outport  Port=3
  wires:
  Gain1/1 -> Gain/1
  In1/1 -> Product18/2, Square/1
  Constant1/1 -> Product2/1
  Cos1/1 -> Product2/2
  Product2/1 -> Product3/1
  Gain/1 -> Product10/2, Product11/2, Product3/2
  In6/1 -> Product4/1, Product13/2, Product12/2
  In7/1 -> Product4/2
  Product3/1 -> Product5/2
  Sin1/1 -> Product6/2
  Product6/1 -> Product10/1
  Constant2/1 -> Product6/1
  Constant3/1 -> Product8/1
  Sin2/1 -> Product8/2
  Product8/1 -> Product11/1
  Product9/1 -> Product15/2
  Product11/1 -> Product9/1
  Product10/1 -> Product7/1
  Product4/1 -> Product5/1
  In8/1 -> Product12/1, Square2/1
  Product12/1 -> Product7/2
  Square2/1 -> Product13/1
  Product13/1 -> Product9/2
  Square/1 -> Gain1/1
  Gain2/1 -> Sin2/1
  Sum1/1 -> Sum4/2
  Sum2/1 -> Product14/1
  Product1/1 -> Sum7/1
  Mod1/1 -> Sum5/1, Sum1/2, Less Than/1, GreaterThan/1
  Sum5/1 -> Sum2/2
  Constant7/1 -> Mod1/2
  Less Than/1 -> Product14/2
  Constant8/1 -> Sum2/1, Sum4/1
  Degrees to Radians2/1 -> Sum6/1
  In2/1 -> Degrees to Radians2/1
  GreaterThan/1 -> Product1/2
  Sum6/1 -> Mod1/1
  Constant5/1 -> Sum6/2
  In5/1 -> Less Than/2, GreaterThan/2, Sum5/2, Sum1/1
  Constant4/1 -> Sum6/3
  Product14/1 -> Sum7/2
  Sum4/1 -> Product1/1
  Sum7/1 -> Gain2/1, Cos1/1, Sin1/1
  Ramp/1 -> Saturation/1
  Product15/1 -> Scope/1, Out5/1
  Product5/1 -> Product17/2
  Product7/1 -> Product16/2
  Product17/1 -> Scope/3, Out3/1
  Saturation/1 -> Transfer Fcn/1
  Transfer Fcn/1 -> Product18/1, Product17/1, Product16/1, Product15/1
  Product16/1 -> Scope/2, Out4/1
  Product18/1 -> To Workspace/1
